simulink model "monitor"  (Simulink 7.7)
settings: Solver=FixedStepDiscrete  StartTime=0.0  StopTime=inf  FixedStep=1  RelTol=1e-3
InitFcn:
  | initMonitor;
values from neighbouring files (symbols this model uses):
  nj = 25    [initCompleteForceControlSim.m]    (also in initMonitor.m; initMonitorSim.m; initPartialForceControl.m; initPartialForceControlSim.m)
  Rf = [R, zeros(3,3); zeros(3,3), R]    [initBalancingControllerWithHandControl.m]    (also in initCompleteForceControlSim.m; initMonitor.m; initMonitorSim.m; initPartialForceControl.m)
libraries: WBCLibrary x11, simulink x2, dspsigops x2
settings Model: Creator=daniele  LastModifiedBy=iron
settings DataIOCC: SignalLoggingSaveFormat=Dataset
settings DebuggingCC: FcnCallInpInsideContextMsg=Enable All

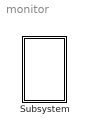
== system monitor ==
  Subsystem : Subsystem  mask{robotName='icub', Ts=0.01, localName='dynamicBalancing'}
      mask prompts: robotName "robot name"; localName "module name"

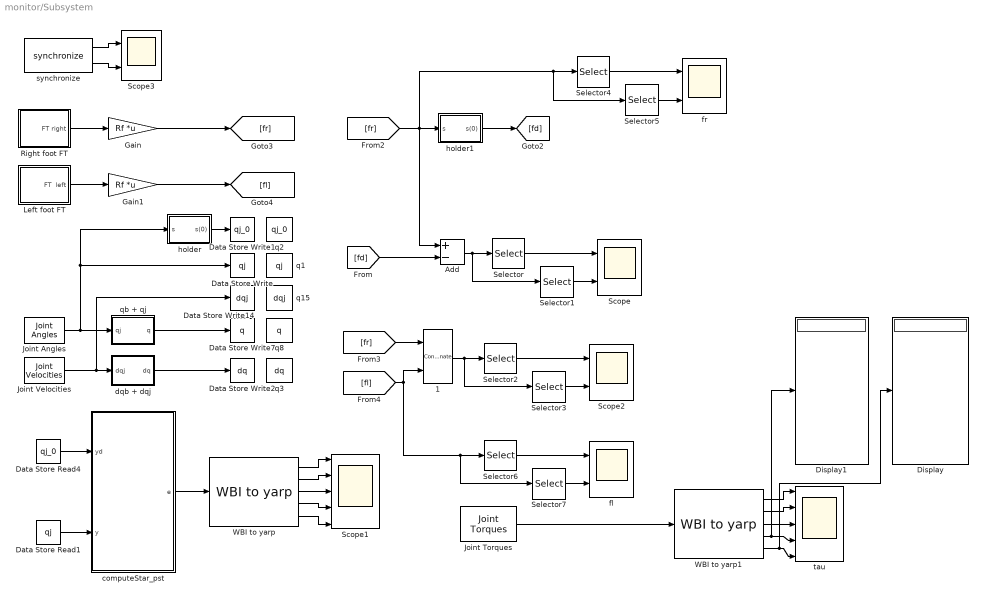
== system monitor/Subsystem ==
  " 1" : Concatenate  Mode=Multidimensional array
  Add : Sum  Inputs=+-
  Data Store Read1 : DataStoreRead  DataStoreName=qj
  Data Store Read4 : DataStoreRead  DataStoreName=qj_0
  Data Store Write : DataStoreWrite  Priority=-1  DataStoreName=qj
  Data Store Write1 : DataStoreWrite  Priority=-1  DataStoreName=qj_0
  Data Store Write14 : DataStoreWrite  Priority=-1  DataStoreName=dqj
  Data Store Write2 : DataStoreWrite  Priority=-1  DataStoreName=dq
  Data Store Write7 : DataStoreWrite  Priority=-1  DataStoreName=q
  Display : Display
  Display1 : Display
  Gain : Gain  Gain=Rf  Multiplication=Matrix(K*u)
  Gain1 : Gain  Gain=Rf  Multiplication=Matrix(K*u)
  Joint Angles : WBCLibrary/wholeBodyStates/Joint Angles  SystemSampleTime=-1  robotName=robotName  localName=localName
  Joint Torques : WBCLibrary/wholeBodyStates/Joint Torques  SystemSampleTime=-1  robotName=robotName  localName=localName
  Joint Velocities : WBCLibrary/wholeBodyStates/Joint Velocities  SystemSampleTime=-1  robotName=robotName  localName=localName
  Left foot FT : Subsystem
  Right foot FT : Subsystem
  Scope : Scope  NumInputPorts=2
      settings: TimeRange=1200  YMin=-9.5~-5  YMax=2~1.5
  Scope1 : Scope  NumInputPorts=5
      settings: TimeRange=2000  YMin=-0.45~-0.3~-0.2~-0.4~-0.5  YMax=2.77556e-17~0.5~0.25~0.4~0.2
  Scope2 : Scope  NumInputPorts=2
      settings: TimeRange=1200  YMin=-10~-2.75  YMax=120~0.25  SaveName=ScopeData2
  Scope3 : Scope  NumInputPorts=2
      settings: TimeRange=1200  YMin=-14~-5  YMax=6~5  SaveName=ScopeData3
  Selector : Selector  InputPortWidth=6  IndexOptions=Index vector (dialog)  Indices=[1:3]  OutputSizes=1
  Selector1 : Selector  InputPortWidth=6  IndexOptions=Index vector (dialog)  Indices=[4:6]  OutputSizes=1
  Selector2 : Selector  InputPortWidth=12  IndexOptions=Index vector (dialog)  Indices=[1:3 7:9]  OutputSizes=1
  Selector3 : Selector  InputPortWidth=12  IndexOptions=Index vector (dialog)  Indices=[4:6 10:12]  OutputSizes=1
  Selector4 : Selector  InputPortWidth=6  IndexOptions=Index vector (dialog)  Indices=[1:3]  OutputSizes=1
  Selector5 : Selector  InputPortWidth=6  IndexOptions=Index vector (dialog)  Indices=[4:6]  OutputSizes=1
  Selector6 : Selector  InputPortWidth=6  IndexOptions=Index vector (dialog)  Indices=[1:3]  OutputSizes=1
  Selector7 : Selector  InputPortWidth=6  IndexOptions=Index vector (dialog)  Indices=[4:6]  OutputSizes=1
  WBI to yarp : WBCLibrary/Utilities/WBI to yarp  SystemSampleTime=-1
  WBI to yarp1 : WBCLibrary/Utilities/WBI to yarp  SystemSampleTime=-1
  computeStar_pst : Subsystem
  dqb + dqj : Subsystem
  fl : Scope  NumInputPorts=2
      settings: TimeRange=1800  YMin=-30~-2.25  YMax=170~3.5  SaveName=ScopeData5
  fr : Scope  NumInputPorts=2
      settings: TimeRange=1800  YMin=-50~-16  YMax=170~3  SaveName=ScopeData4
  holder : Subsystem
  holder1 : Subsystem
  q1 : DataStoreMemory  Priority=-1  DataStoreName=qj  ReadBeforeWriteMsg=warning  WriteAfterWriteMsg=warning  WriteAfterReadMsg=warning  InitialValue=zeros(nj,1)  VectorParams1D=off  OutDataTypeStr=double
  q15 : DataStoreMemory  Priority=-1  DataStoreName=dqj  ReadBeforeWriteMsg=warning  WriteAfterWriteMsg=warning  WriteAfterReadMsg=warning  InitialValue=zeros(nj,1)  VectorParams1D=off  OutDataTypeStr=double
  q2 : DataStoreMemory  Priority=-1  DataStoreName=qj_0  ReadBeforeWriteMsg=warning  WriteAfterWriteMsg=warning  WriteAfterReadMsg=warning  InitialValue=zeros(nj,1)  VectorParams1D=off  OutDataTypeStr=double
  q3 : DataStoreMemory  Priority=-1  DataStoreName=dq  ReadBeforeWriteMsg=warning  WriteAfterWriteMsg=warning  WriteAfterReadMsg=warning  InitialValue=zeros(nj+6,1)  VectorParams1D=off  OutDataTypeStr=double
  q8 : DataStoreMemory  Priority=-1  DataStoreName=q  ReadBeforeWriteMsg=warning  WriteAfterWriteMsg=warning  WriteAfterReadMsg=warning  InitialValue=zeros(nj+16,1)  VectorParams1D=off  OutDataTypeStr=double
  qb + qj : Subsystem
  synchronize : WBCLibrary/Utilities/synchronize  rate=0.010  scaleFactor=1
  tau : Scope  NumInputPorts=5
      settings: TimeRange=2000  YMin=-12.5~-1.5~-1.5~-8~-6  YMax=2.5~1.5~1.5~6~8  SaveName=ScopeData6
  wires:
  qb + qj/1(q) -> Data Store Write7/1
  dqb + dqj/1(dq) -> Data Store Write2/1
  holder/1(s(0)) -> Data Store Write1/1
  Joint Velocities/1 -> dqb + dqj/1(dqj), Data Store Write14/1
  Joint Angles/1 -> qb + qj/1(qj), Data Store Write/1, holder/1(s)
  Data Store Read1/1 -> computeStar_pst/2(y)
  WBI to yarp/1 -> Scope1/1
  WBI to yarp/2 -> Scope1/2
  WBI to yarp/3 -> Scope1/3
  WBI to yarp/4 -> Scope1/4
  WBI to yarp/5 -> Scope1/5
  [fr] -> holder1/1(s), Add/1, Selector4/1, Selector5/1
  holder1/1(s(0)) -> [fd]
  [fd] -> Add/2
  Add/1 -> Selector/1, Selector1/1
  Selector/1 -> Scope/1
  Selector1/1 -> Scope/2
  computeStar_pst/1(e) -> WBI to yarp/1
  Right foot FT/1(FT right) -> Gain/1
  Left foot FT/1(FT  left) -> Gain1/1
  " 1"/1 -> Selector2/1, Selector3/1
  Selector2/1 -> Scope2/1
  Selector3/1 -> Scope2/2
  [fr] -> " 1"/1
  [fl] -> " 1"/2, Selector6/1, Selector7/1
  Data Store Read4/1 -> computeStar_pst/1(yd)
  synchronize/1 -> Scope3/1
  synchronize/2 -> Scope3/2
  Selector4/1 -> fr/1
  Selector5/1 -> fr/2
  Selector6/1 -> fl/1
  Selector7/1 -> fl/2
  Gain/1 -> [fr]
  Gain1/1 -> [fl]
  WBI to yarp1/1 -> tau/1
  WBI to yarp1/2 -> tau/2
  WBI to yarp1/3 -> tau/3
  WBI to yarp1/4 -> tau/4, Display1/1
  WBI to yarp1/5 -> tau/5, Display/1
  Joint Torques/1 -> WBI to yarp1/1

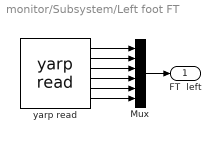
== system monitor/Subsystem/Left foot FT ==
  Mux : Mux  Inputs=6
  yarp read : WBCLibrary/Utilities/yarp read  from='/wholeBodyDyanmicsTree/left_leg/endEffectorWrench:o'  to='...'  num=6
  FT  left : Outport
  wires:
  yarp read/1 -> Mux/1
  yarp read/2 -> Mux/2
  yarp read/3 -> Mux/3
  yarp read/4 -> Mux/4
  yarp read/5 -> Mux/5
  yarp read/6 -> Mux/6
  Mux/1 -> FT  left/1

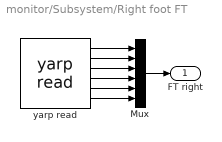
== system monitor/Subsystem/Right foot FT ==
  Mux : Mux  Inputs=6
  yarp read : WBCLibrary/Utilities/yarp read  from='/wholeBodyDyanmicsTree/right_leg/endEffectorWrench:o'  to='...'  num=6
  FT right : Outport
  wires:
  yarp read/1 -> Mux/1
  yarp read/2 -> Mux/2
  yarp read/3 -> Mux/3
  yarp read/4 -> Mux/4
  yarp read/5 -> Mux/5
  yarp read/6 -> Mux/6
  Mux/1 -> FT right/1

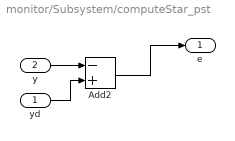
== system monitor/Subsystem/computeStar_pst ==
  yd : Inport
  y : Inport  Port=2
  Add2 : Sum  Inputs=-+
  e : Outport
  wires:
  yd/1 -> Add2/2
  Add2/1 -> e/1
  y/1 -> Add2/1

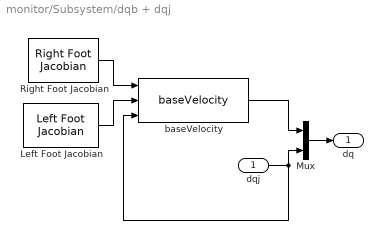
== system monitor/Subsystem/dqb + dqj ==
  dqj : Inport
  Left Foot Jacobian : WBCLibrary/wholeBodyModel/Jacobians/Left Foot Jacobian  SystemSampleTime=-1  robotName=robotName  localName=localName
  Mux : Mux  Inputs=2
  Right Foot Jacobian : WBCLibrary/wholeBodyModel/Jacobians/Right Foot Jacobian  SystemSampleTime=-1  robotName=robotName  localName=localName
  baseVelocity : WBCLibrary/Utilities/baseVelocity  SystemSampleTime=-1
  dq : Outport
  wires:
  Left Foot Jacobian/1 -> baseVelocity/2
  Right Foot Jacobian/1 -> baseVelocity/1
  baseVelocity/1 -> Mux/1
  dqj/1 -> baseVelocity/3, Mux/2
  Mux/1 -> dq/1

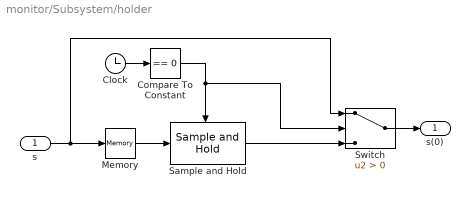
== system monitor/Subsystem/holder ==
  s : Inport
  Clock : Clock
      settings: Decimation=10
  Compare To Constant : simulink/Logic and Bit Operations/Compare To Constant  SystemSampleTime=-1  relop===  const=0  LogicOutDataTypeMode=boolean
  Memory : Memory
  Sample and Hold : dspsigops/Sample and Hold  SystemSampleTime=-1  trig=Falling edge  initCond=0  latchinput=off
  Switch : Switch  Criteria=u2 > Threshold
  s(0) : Outport
  wires:
  s/1 -> Switch/1, Memory/1
  Clock/1 -> Compare To Constant/1
  Compare To Constant/1 -> Sample and Hold/Trigger, Switch/2
  Sample and Hold/1 -> Switch/3
  Switch/1 -> s(0)/1
  Memory/1 -> Sample and Hold/1

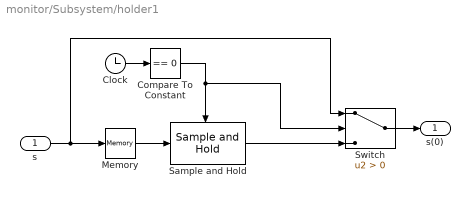
== system monitor/Subsystem/holder1 ==
  s : Inport
  Clock : Clock
      settings: Decimation=10
  Compare To Constant : simulink/Logic and Bit Operations/Compare To Constant  SystemSampleTime=-1  relop===  const=0  LogicOutDataTypeMode=boolean
  Memory : Memory
  Sample and Hold : dspsigops/Sample and Hold  SystemSampleTime=-1  trig=Falling edge  initCond=0  latchinput=off
  Switch : Switch  Criteria=u2 > Threshold
  s(0) : Outport
  wires:
  Memory/1 -> Sample and Hold/1
  Switch/1 -> s(0)/1
  Sample and Hold/1 -> Switch/3
  Compare To Constant/1 -> Switch/2, Sample and Hold/Trigger
  Clock/1 -> Compare To Constant/1
  s/1 -> Memory/1, Switch/1

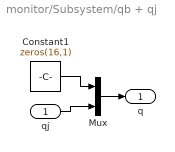
== system monitor/Subsystem/qb + qj ==
  qj : Inport
  Constant1 : Constant  Value=zeros(16,1)
  Mux : Mux  Inputs=2
  q : Outport
  wires:
  Mux/1 -> q/1
  Constant1/1 -> Mux/1
  qj/1 -> Mux/2
